simulink model "newattempt01"  (R2020a)
settings: Solver=FixedStepAuto  StartTime=0.0  StopTime=0.02  FixedStep=0.00001  RelTol=1e-3
model workspace (MAT data in the model file):
  K_Spring = 3
  R = 7
  V = 350
  V_T = Simulink.Parameter
  V_T.Value = 350
  V_T.DataType = 'auto'
  V_T.Dimensions = [1 1]
libraries: nesl_utility x27, fl_lib x21, sdl_lib x1
settings Model: OrderedModelArguments=off  Creator=insat  LastModifiedBy=insat

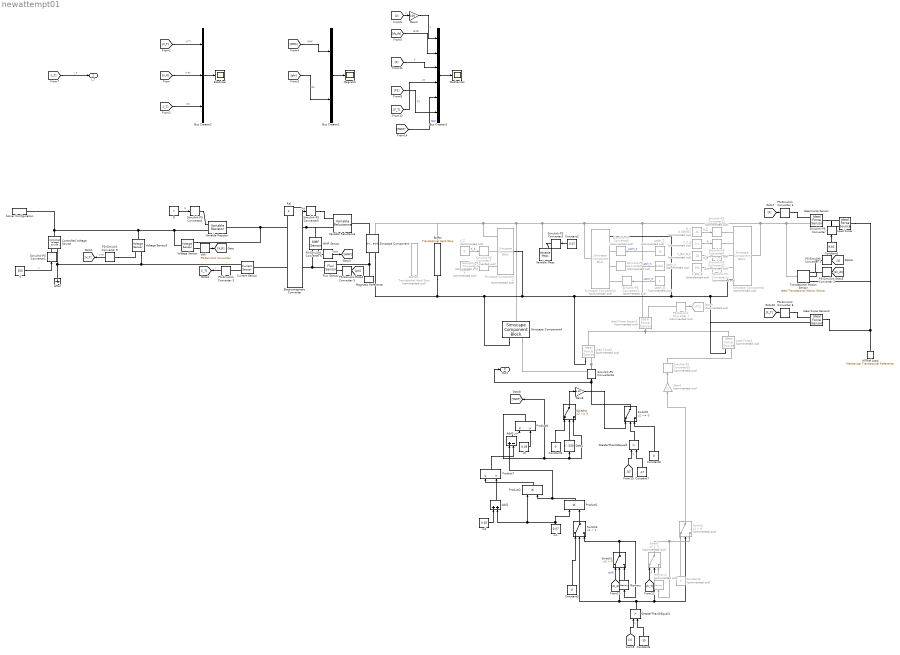
== system newattempt01 ==
  Add1 : Sum
  Add2 : Sum  Inputs=+-
  Buffer : fl_lib/Mechanical/Translational Elements/Translational Hard Stop  upper_bnd=20 mm  lower_bnd=-.9 mm  stiff_up=100 N/mm  stiff_low=100 N/mm  D_up=100 s*N/mm  D_low=100 s*N/mm  model=simscape.enum.hardstop.fullundamped  transition=1 mm  v_specify=off  v_priority=None  v=0 m/s  v_nominal_specify=off  v_nominal_unit=m/s  v_nominal_value=1  f_specify=off  f_priority=None  f=0 N  f_nominal_specify=off  f_nominal_unit=N  f_nominal_value=1  x_specify=off  x_priority=High  x=0 m  x_nominal_specify=off  x_nominal_unit=m  x_nominal_value=1
  Buffer1 : fl_lib/Mechanical/Translational Elements/Translational Hard Stop  Commented=on  upper_bnd=20 mm  lower_bnd=-.9 mm  stiff_up=10000 N/mm  stiff_low=10000 N/mm  D_up=0.7 s*N/mm  D_low=0.7 s*N/mm  model=simscape.enum.hardstop.fullundamped  transition=1 mm  v_specify=off  v_priority=None  v=0 m/s  v_nominal_specify=off  v_nominal_unit=m/s  v_nominal_value=1  f_specify=off  f_priority=None  f=0 N  f_nominal_specify=off  f_nominal_unit=N  f_nominal_value=1  x_specify=off  x_priority=High  x=0 m  x_nominal_specify=off  x_nominal_unit=m  x_nominal_value=1
  Bus Creator1 : BusCreator  Inputs=2
  Bus Creator2 : BusCreator  Inputs=3
  Bus Creator3 : BusCreator  Inputs=6
  Constant1 : Constant  Value=9.81
  Constant2 : Constant  Value=0.07
  Constant3 : Constant  Commented=on  Value=0
  Constant4 : Constant  Value=-15
  Constant5 : Constant  Value=0
  Constant6 : Constant  Value=0
  Constant7 : Constant  Value=-17
  Constant8 : Constant  Value=0
  Controlled Voltage Source : fl_lib/Electrical/Electrical Sources/Controlled Voltage Source
  Current Sensor : fl_lib/Electrical/Electrical Sensors/Current Sensor
  D_V : Constant  Commented=on  Value=0.000001
  Delay : Delay  DelayLength=250  InitialCondition=0  UseCircularBuffer=on
  ERef : fl_lib/Electrical/Electrical Elements/Electrical Reference
  Electrical : Scope
  Electromagnetic Converter : fl_lib/Magnetic/Magnetic Elements/Electromagnetic Converter  Nw=1000  i_specify=off  i_priority=None  i=0 A  i_nominal_specify=off  i_nominal_unit=A  i_nominal_value=1  v_specify=off  v_priority=None  v=0 V  v_nominal_specify=off  v_nominal_unit=V  v_nominal_value=1  mmf_specify=off  mmf_priority=None  mmf=0 A  mmf_nominal_specify=off  mmf_nominal_unit=A  mmf_nominal_value=1  phi_specify=off  phi_priority=High  phi=0 Wb  phi_nominal_specify=off  phi_nominal_unit=Wb  phi_nominal_value=1
      settings: SourceProductBaseCode=SS  InternalSimscapePortConfiguration="{\"Bottom\":[],\"Left\":[{\"id\":\"p\",\"label\":\"+\",\"type\":\"foundation.electrical.electrical\"},{\"id\":\"n\",\"label\":\"-\",\"type\":\"foundation.electrical.electrical\"}],\"Right\":[{\"id\":\"N\",\"label\":\"N\",\"type\":\"foundation.magnetic.magnetic\"},{\"id\":\"S\",\"label\":\"S\",\"type\":\"foundation.magnetic.magnetic\"}],\"Top\":[]}"
  F_BW_B : Constant  Commented=on  Value=250
  F_C_B : Constant  Commented=on  Value=0.1
  Flux Sensor : fl_lib/Magnetic/Magnetic Sensors/Flux Sensor
      settings: SourceProductBaseCode=SS  InternalSimscapePortConfiguration="{\"Bottom\":[],\"Left\":[{\"id\":\"N\",\"label\":\"N\",\"type\":\"foundation.magnetic.magnetic\"}],\"Right\":[{\"id\":\"PHI\",\"label\":\"\",\"type\":\"output\"},{\"id\":\"S\",\"label\":\"S\",\"type\":\"foundation.magnetic.magnetic\"}],\"Top\":[]}"
  Gain2 : Gain  Gain=100
  Gain3 : Gain  Gain=-0.05
  Gain4 : Gain  Commented=on  Gain=-1
  Goto9 : Goto  Commented=on  GotoTag=F2
  GreaterThanOrEqual1 : RelationalOperator  Operator=>  OutDataTypeStr=boolean  ZeroCross=off  RndMeth=Simplest
  GreaterThanOrEqual2 : RelationalOperator  Operator=>  OutDataTypeStr=boolean  ZeroCross=off  RndMeth=Simplest
  Ideal Force Sensor : fl_lib/Mechanical/Mechanical Sensors/Ideal Force Sensor
  Ideal Force Sensor1 : fl_lib/Mechanical/Mechanical Sensors/Ideal Force Sensor  Commented=on
  Ideal Force Sensor2 : fl_lib/Mechanical/Mechanical Sensors/Ideal Force Sensor
  K : Constant  Commented=on  Value=3
  K_Z : Constant  Commented=on  Value=0
  Latch_D : Constant  Commented=on
  Latch_K : Constant  Commented=on  Value=0.0001
  Latch_Z : Constant  Commented=on  Value=15
  Load Force : fl_lib/Mechanical/Mechanical Sources/Ideal Force Source
  Load Force1 : fl_lib/Mechanical/Mechanical Sources/Ideal Force Source  Commented=on
  Load Force2 : fl_lib/Mechanical/Mechanical Sources/Ideal Force Source  Commented=on
  MMF Sensor : fl_lib/Magnetic/Magnetic Sensors/MMF Sensor
      settings: SourceProductBaseCode=SS  InternalSimscapePortConfiguration="{\"Bottom\":[],\"Left\":[{\"id\":\"N\",\"label\":\"N\",\"type\":\"foundation.magnetic.magnetic\"}],\"Right\":[{\"id\":\"MMF\",\"label\":\"\",\"type\":\"output\"},{\"id\":\"S\",\"label\":\"S\",\"type\":\"foundation.magnetic.magnetic\"}],\"Top\":[]}"
  MTRef Load : fl_lib/Mechanical/Translational Elements/Mechanical Translational Reference
  Magnetic : Scope
  Magnetic Reference : fl_lib/Magnetic/Magnetic Elements/Magnetic Reference
      settings: SourceProductBaseCode=SS  InternalSimscapePortConfiguration="{\"Bottom\":[],\"Left\":[{\"id\":\"M\",\"label\":\"\",\"type\":\"foundation.magnetic.magnetic\"}],\"Right\":[],\"Top\":[]}"
  Mechanical : Scope
  Memory : Memory
  Memory1 : Memory  Commented=on
  PS-Simulink Converter 1 : nesl_utility/PS-Simulink Converter  PhysicalDomain=network_engine_domain  SubClassName=ps_output  LeftPortType=input  RightPortType=output  PseudoPeriodic=off  Frequencies=[]  Unit=mm  AffineConversion=off
  PS-Simulink Converter 2 : nesl_utility/PS-Simulink Converter  PhysicalDomain=network_engine_domain  SubClassName=ps_output  LeftPortType=input  RightPortType=output  PseudoPeriodic=off  Frequencies=[]  Unit=mm/s  AffineConversion=off
  PS-Simulink Converter 3 : nesl_utility/PS-Simulink Converter  PhysicalDomain=network_engine_domain  SubClassName=ps_output  LeftPortType=input  RightPortType=output  PseudoPeriodic=off  Frequencies=[]  Unit=A  AffineConversion=off
  PS-Simulink Converter 4 : nesl_utility/PS-Simulink Converter  PhysicalDomain=network_engine_domain  SubClassName=ps_output  LeftPortType=input  RightPortType=output  PseudoPeriodic=off  Frequencies=[]  Unit=N  AffineConversion=off
  PS-Simulink Converter 5 : nesl_utility/PS-Simulink Converter  PhysicalDomain=network_engine_domain  SubClassName=ps_output  LeftPortType=input  RightPortType=output  PseudoPeriodic=off  Frequencies=[]  Unit=Wb  AffineConversion=off
  PS-Simulink Converter 6 : nesl_utility/PS-Simulink Converter  PhysicalDomain=network_engine_domain  SubClassName=ps_output  LeftPortType=input  RightPortType=output  PseudoPeriodic=off  Frequencies=[]  Unit=A  AffineConversion=off
  PS-Simulink Converter 7 : nesl_utility/PS-Simulink Converter  Commented=on  PhysicalDomain=network_engine_domain  SubClassName=ps_output  LeftPortType=input  RightPortType=output  PseudoPeriodic=off  Frequencies=[]  Unit=N  AffineConversion=off
  PS-Simulink Converter 8 : nesl_utility/PS-Simulink Converter  PhysicalDomain=network_engine_domain  SubClassName=ps_output  LeftPortType=input  RightPortType=output  PseudoPeriodic=off  Frequencies=[]  Unit=N  AffineConversion=off
  PS-Simulink Converter 9 : nesl_utility/PS-Simulink Converter  PhysicalDomain=network_engine_domain  SubClassName=ps_output  LeftPortType=input  RightPortType=output  PseudoPeriodic=off  Frequencies=[]  Unit=V  AffineConversion=off
  Product1 : Product  Inputs=**
  Product2 : Product  Inputs=**
  Product7 : Product  Inputs=*/
  Product8 : Product  Inputs=*/
  R : Constant  Value=7
  Rel : Constant
  Simscape Component : SimscapeComponentBlock  SourceFile=reluctance_force_actuator_modified  ComponentPath=reluctance_force_actuator_modified  ComponentVariants="[\"reluctance_force_actuator_modified\"]"  ComponentVariantNames="[\"reluctance_force_actuator_modified\"]"  ClassName=reluctance_force_actuator_modified  SchemaVersion=1  x0=30 mm  xbffr=1 mm  CSA=1.7671 cm^2  mur=1  K_contact=500 N/mm  D_contact=0.2 s*N/mm  mmf_specify=off  mmf_priority=None  mmf=0 A  mmf_nominal_specify=off  mmf_nominal_unit=A  mmf_nominal_value=1  phi_specify=off  phi_priority=None  phi=0 Wb  phi_nominal_specify=off  phi_nominal_unit=Wb  phi_nominal_value=1  f_specify=off  f_priority=None  f=0 N  f_nominal_specify=off  f_nominal_unit=N  f_nominal_value=1  u_specify=off  u_priority=None  u=0 m/s  u_nominal_specify=off  u_nominal_unit=m/s  u_nominal_value=1
      settings: CopyFcn=simscape.engine.sli.internal.componentblockcallback(gcbh,'COPY')  PreCopyFcn=simscape.engine.sli.internal.componentblockcallback(gcbh,'PRECOPY')  PreDeleteFcn=simscape.engine.sli.internal.componentblockcallback(gcbh,'PREDELETE')  InternalSimscapePortConfiguration="{\"Bottom\":[],\"Left\":[{\"id\":\"N\",\"label\":\"N\",\"type\":\"foundation.magnetic.magnetic\"},{\"id\":\"R\",\"label\":\"R\",\"type\":\"foundation.mechanical.translational.translational\"}],\"Right\":[{\"id\":\"S\",\"label\":\"S\",\"type\":\"foundation.magnetic.magnetic\"},{\"id\":\"C\",\"label\":\"C\",\"type\":\"foundation.mechanical.translational.translational\"}],\"Top\":[]}"
      mask Type: Reluctance Force Actuator
  Simscape Component1 : SimscapeComponentBlock  Commented=on  SourceFile=mechanical_forces_from_reluctance_force_actuator  ComponentPath=mechanical_forces_from_reluctance_force_actuator  ComponentVariants="[\"mechanical_forces_from_reluctance_force_actuator\"]"  ComponentVariantNames="[\"mechanical_forces_from_reluctance_force_actuator\"]"  ClassName=mechanical_forces_from_reluctance_force_actuator  SchemaVersion=1  latch_dur=1 mm  transition=0.1 mm  v_specify=off  v_priority=None  v=0 m/s  v_nominal_specify=off  v_nominal_unit=m/s  v_nominal_value=1  f_specify=off  f_priority=None  f=0 N  f_nominal_specify=off  f_nominal_unit=N  f_nominal_value=1  x_specify=off  x_priority=High  x=0 m  x_nominal_specify=off  x_nominal_unit=m  x_nominal_value=1
      settings: CopyFcn=simscape.engine.sli.internal.componentblockcallback(gcbh,'COPY')  PreCopyFcn=simscape.engine.sli.internal.componentblockcallback(gcbh,'PRECOPY')  PreDeleteFcn=simscape.engine.sli.internal.componentblockcallback(gcbh,'PREDELETE')  InternalSimscapePortConfiguration="{\"Bottom\":[],\"Left\":[{\"id\":\"R\",\"label\":\"R\",\"type\":\"foundation.mechanical.translational.translational\"},{\"id\":\"latch_loc\",\"label\":\"Z\",\"type\":\"input\"},{\"id\":\"K_latch\",\"label\":\"K\",\"type\":\"input\"},{\"id\":\"D_latch\",\"label\":\"D\",\"type\":\"input\"}],\"Right\":[{\"id\":\"C\",\"label\":\"C\",\"type\":\"foundation.mechanical.translational.translational\"}],\"Top\":[]}"
      mask Type: Mechanical Forces from Reluctance Force Actuator
  Simscape Component2 : SimscapeComponentBlock  Commented=on  SourceFile=var_trans_spring_mod  ComponentPath=var_trans_spring_mod  ComponentVariants="[\"var_trans_spring_mod\"]"  ComponentVariantNames="[\"var_trans_spring_mod\"]"  ClassName=var_trans_spring_mod  SchemaVersion=1  Kmin=1 N/m
      settings: CopyFcn=simscape.engine.sli.internal.componentblockcallback(gcbh,'COPY')  PreCopyFcn=simscape.engine.sli.internal.componentblockcallback(gcbh,'PRECOPY')  PreDeleteFcn=simscape.engine.sli.internal.componentblockcallback(gcbh,'PREDELETE')  InternalSimscapePortConfiguration="{\"Bottom\":[],\"Left\":[{\"id\":\"R\",\"label\":\"R\",\"type\":\"foundation.mechanical.translational.translational\"}],\"Right\":[{\"id\":\"K\",\"label\":\"K\",\"type\":\"input\"},{\"id\":\"Z\",\"label\":\"Z\",\"type\":\"input\"},{\"id\":\"C\",\"label\":\"C\",\"type\":\"foundation.mechanical.translational.translational\"}],\"Top\":[]}"
      mask Type: Variable Translational Spring
  Simscape Component3 : SimscapeComponentBlock  Commented=on  SourceFile=friction_var  ComponentPath=friction_var  ComponentVariants="[\"friction_var\"]"  ComponentVariantNames="[\"friction_var\"]"  ClassName=friction_var  SchemaVersion=1  v_specify=off  v_priority=None  v=0 m/s  v_nominal_specify=off  v_nominal_unit=m/s  v_nominal_value=1  f_specify=off  f_priority=None  f=0 N  f_nominal_specify=off  f_nominal_unit=N  f_nominal_value=1
      settings: CopyFcn=simscape.engine.sli.internal.componentblockcallback(gcbh,'COPY')  PreCopyFcn=simscape.engine.sli.internal.componentblockcallback(gcbh,'PRECOPY')  PreDeleteFcn=simscape.engine.sli.internal.componentblockcallback(gcbh,'PREDELETE')  InternalSimscapePortConfiguration="{\"Bottom\":[],\"Left\":[{\"id\":\"R\",\"label\":\"R\",\"type\":\"foundation.mechanical.translational.translational\"},{\"id\":\"brkwy_frc\",\"label\":\"F_BW_B\",\"type\":\"input\"},{\"id\":\"brkwy_vel\",\"label\":\"V_BW_B\",\"type\":\"input\"},{\"id\":\"Col_frc\",\"label\":\"F_C_B\",\"type\":\"input\"},{\"id\":\"visc_coef\",\"label\":\"D_V\",\"type\":\"input\"}],\"Right\":[{\"id\":\"C\",\"label\":\"C\",\"type\":\"foundation.mechanical.translational.translational\"}],\"Top\":[]}"
      mask Type: Translational Friction Controllable
  Simscape Component4 : SimscapeComponentBlock  SourceFile=damper_mod  ComponentPath=damper_mod  ComponentVariants="[\"damper_mod\"]"  ComponentVariantNames="[\"damper_mod\"]"  ClassName=damper_mod  SchemaVersion=1  v_specify=off  v_priority=None  v=0 m/s  v_nominal_specify=off  v_nominal_unit=m/s  v_nominal_value=1  f_specify=off  f_priority=None  f=0 N  f_nominal_specify=off  f_nominal_unit=N  f_nominal_value=1
      settings: CopyFcn=simscape.engine.sli.internal.componentblockcallback(gcbh,'COPY')  PreCopyFcn=simscape.engine.sli.internal.componentblockcallback(gcbh,'PRECOPY')  PreDeleteFcn=simscape.engine.sli.internal.componentblockcallback(gcbh,'PREDELETE')  InternalSimscapePortConfiguration="{\"Bottom\":[],\"Left\":[{\"id\":\"R\",\"label\":\"R\",\"type\":\"foundation.mechanical.translational.translational\"},{\"id\":\"D\",\"label\":\"Damping coefficient\",\"type\":\"input\"}],\"Right\":[{\"id\":\"C\",\"label\":\"C\",\"type\":\"foundation.mechanical.translational.translational\"}],\"Top\":[]}"
      mask Type: Translational Damper
  Simulink-PS Converter{,1,3..5,16} (6 alike) : nesl_utility/Simulink-PS Converter  PhysicalDomain=network_engine_domain  SubClassName=ps_input  LeftPortType=input  RightPortType=output  PseudoPeriodic=off  Frequencies=[]  NoiseDistribution=none  NoiseParameters=[]  Unit=1  AffineConversion=off  FilteringAndDerivatives=zero  SimscapeFilterOrder=1  InputFilterTimeConstant=.001  UdotUserProvided=0
  Simulink-PS Converter{2,6..13,15} (10 alike) : nesl_utility/Simulink-PS Converter  Commented=on  PhysicalDomain=network_engine_domain  SubClassName=ps_input  LeftPortType=input  RightPortType=output  PseudoPeriodic=off  Frequencies=[]  NoiseDistribution=none  NoiseParameters=[]  Unit=1  AffineConversion=off  FilteringAndDerivatives=zero  SimscapeFilterOrder=1  InputFilterTimeConstant=.001  UdotUserProvided=0
  Solver Configuration : nesl_utility/Solver Configuration  PhysicalDomain=network_engine_domain  SubClassName=solver  LeftPortType=input  RightPortType=generic  Tones=[]  Harmonics=[]  SimulateNoise=off  Profile=off  UseLocalSampling=off  EnableSwitchedLinearOptims=on  FrequencyDomain=off  UseCCode=off  RelTol=0.001  AbsTol=1e-06  MinStep=1e-09  ToWorkspace=off  RevertToSquareIcSolve=off  NumHomotopyIterations=100  PhasorMode=off  PhasorModeNumHarmonics=1  DoDC=off  ResidualTolerance=1e-9  UseLocalSolver=off  LocalSolverChoice=NE_BACKWARD_EULER_ADVANCER  LocalSolverSampleTime=.001  DoFixedCost=off  MaxNonlinIter=3  MaxModeIter=2  LinearAlgebra=auto  EquationFormulation=NE_TIME_EF  DelaysMemoryBudget=1024  AutomaticFiltering=on  FilteringTimeConstant=0.0001  PartitionStorageMethod=AS_NEEDED  PartitionMemoryBudget=1024  PartitionMethod=FAST
  Switch : Switch  Commented=on  Criteria=u2 > Threshold
  Switch1 : Switch  Criteria=u2 > Threshold
  Switch2 : Switch  Commented=on  Criteria=u2 > Threshold
  Switch3 : Switch  Criteria=u2 > Threshold
  Switch4 : Switch  Criteria=u2 ~= 0  ZeroCross=off
  Switch5 : Switch  Criteria=u2 ~= 0  ZeroCross=off
  Translational Motion Sensor : fl_lib/Mechanical/Mechanical Sensors/Ideal Translational Motion Sensor  offset=0 mm
  V : Constant  Value=350
  V(R) : nesl_utility/PS-Simulink Converter  PhysicalDomain=network_engine_domain  SubClassName=ps_output  LeftPortType=input  RightPortType=output  PseudoPeriodic=off  Frequencies=[]  Unit=V  AffineConversion=off
  V_BW_B_C : Constant  Commented=on  Value=10
  Variable Mass : sdl_lib/Inertias & Loads/Variable Mass  minimum_mass=0.0001 kg  p_specify=off  p_priority=High  p=0 m*kg/s  p_nominal_specify=off  p_nominal_unit=m*kg/s  p_nominal_value=1
      settings: SourceProductBaseCode=LD  InternalSimscapePortConfiguration="{\"Bottom\":[],\"Left\":[{\"id\":\"M\",\"label\":\"\",\"type\":\"input\"},{\"id\":\"A\",\"label\":\"\",\"type\":\"foundation.mechanical.translational.translational\"}],\"Right\":[],\"Top\":[]}"
  Variable Reluctance : fl_lib/Magnetic/Magnetic Elements/Variable Reluctance  Xmin=1 m  CSA=1 m^2  mur=1  phi_specify=off  phi_priority=None  phi=0 Wb  phi_nominal_specify=off  phi_nominal_unit=Wb  phi_nominal_value=1  mmf_specify=off  mmf_priority=None  mmf=0 A  mmf_nominal_specify=off  mmf_nominal_unit=A  mmf_nominal_value=1
      settings: SourceProductBaseCode=SS  InternalSimscapePortConfiguration="{\"Bottom\":[],\"Left\":[{\"id\":\"N\",\"label\":\"N\",\"type\":\"foundation.magnetic.magnetic\"},{\"id\":\"X\",\"label\":\"\",\"type\":\"input\"}],\"Right\":[{\"id\":\"S\",\"label\":\"S\",\"type\":\"foundation.magnetic.magnetic\"}],\"Top\":[]}"
  Variable Resistor : fl_lib/Electrical/Electrical Elements/Variable Resistor  Rmin=0 Ohm  i_specify=off  i_priority=None  i=0 A  i_nominal_specify=off  i_nominal_unit=A  i_nominal_value=1  v_specify=off  v_priority=None  v=0 V  v_nominal_specify=off  v_nominal_unit=V  v_nominal_value=1
  Voltage Sensor : fl_lib/Electrical/Electrical Sensors/Voltage Sensor
  Voltage Sensor3 : fl_lib/Electrical/Electrical Sensors/Voltage Sensor
  dt : Constant  Value=0.05
  m1 : Constant  Value=0.07
  m2 : Constant  Value=0.35
  i_T : Outport  SignalName=i_T
  Out1 : Outport  Port=2
  wires:
  PS-Simulink Converter 5/1 -> [phi]
  PS-Simulink Converter 6/1 -> [MMF]  "MMF"
  PS-Simulink Converter 9/1 -> [V_T]  "V(T)"
  PS-Simulink Converter 3/1 -> [i_T]  "i"
  PS-Simulink Converter 1/1 -> [z]
  V(R)/1 -> [V_R]
  PS-Simulink Converter 2/1 -> [dz_dt]
  [V_R] -> Bus Creator2/2  "V(R)"
  [V_T] -> Bus Creator2/1  "V(T)"
  Bus Creator2/1 -> Electrical/1
  [i_T] -> Bus Creator2/3  "i(T)"
  Bus Creator1/1 -> Magnetic/1
  [MMF] -> Bus Creator1/1  "MMF"
  [phi] -> Bus Creator1/2  "phi"
  Bus Creator3/1 -> Mechanical/1
  [z] -> Gain2/1  "z"
  [dz_dt] -> Bus Creator3/2  "dz/dt"
  Constant1/1 -> Simulink-PS Converter/1
  [F] -> Bus Creator3/3  "F"
  Constant2/1 -> Simulink-PS Converter3/1
  K/1 -> Simulink-PS Converter2/1  "K"
  R/1 -> Simulink-PS Converter4/1  "R"
  Rel/1 -> Simulink-PS Converter5/1  "Rel"
  K_Z/1 -> Simulink-PS Converter7/1  "K_Z"
  Latch_Z/1 -> Simulink-PS Converter8/1  "Latch_Z"
  Latch_K/1 -> Simulink-PS Converter9/1  "Latch_K"
  Latch_D/1 -> Simulink-PS Converter10/1  "Latch_D"
  F_C_B/1 -> Simulink-PS Converter6/1  "K"
  D_V/1 -> Simulink-PS Converter11/1  "K_Z"
  F_BW_B/1 -> Simulink-PS Converter13/1  "K"
  V_BW_B_C/1 -> Simulink-PS Converter12/1  "K_Z"
  V/1 -> Simulink-PS Converter1/1  "V"
  [i_T] -> i_T/1  "i_T"
  [F2] -> Bus Creator3/6  "F2"
  Memory/1 -> Switch1/3
  Constant3/1 -> Switch2/1
  Constant4/1 -> GreaterThanOrEqual1/2
  [z] -> GreaterThanOrEqual1/1  "z"
  GreaterThanOrEqual1/1 -> Switch2/2, Switch/2, Switch3/2, Switch1/2
  [F_T] -> Switch/1  "F"
  Constant5/1 -> Switch3/1
  [dz_dt] -> Switch1/1  "dz/dt"
  Memory1/1 -> Switch/3
  Switch1/1 -> Switch3/3, Memory/1
  PS-Simulink Converter 4/1 -> [F]
  Switch/1 -> Memory1/1, Switch2/3
  Switch2/1 -> Gain4/1
  PS-Simulink Converter 7/1 -> Goto9/1
  PS-Simulink Converter 8/1 -> [F_T]
  [F_T] -> Bus Creator3/4  "FT"
  Delay/1 -> Switch4/2
  Constant6/1 -> Switch4/1
  Gain2/1 -> Bus Creator3/1  "z"
  Gain4/1 -> Simulink-PS Converter15/1
  [TEST] -> Bus Creator3/5  "TEST"
  Gain3/1 -> Switch5/1
  Switch4/1 -> Gain3/1
  m1/1 -> Add1/2, Product2/1, Product1/1
  Switch3/1 -> Product1/2
  Product1/1 -> Product2/2, Add2/1
  Product2/1 -> Product7/1
  m2/1 -> Add1/1
  Add1/1 -> Product7/2
  dt/1 -> Product8/2
  Product7/1 -> Add2/2
  Product8/1 -> [TEST], Switch4/3, Delay/1
  Add2/1 -> Product8/1
  Constant7/1 -> GreaterThanOrEqual2/2
  [z] -> GreaterThanOrEqual2/1  "z"
  GreaterThanOrEqual2/1 -> Switch5/2
  Constant8/1 -> Switch5/3
  Switch5/1 -> Out1/1, Simulink-PS Converter16/1
  connections:
  Voltage Sensor/RConn2 -- Variable Resistor/RConn1 -- Electromagnetic Converter/LConn1
  Flux Sensor/RConn2 -- Simscape Component/RConn1 -- Magnetic Reference/LConn1
  Electromagnetic Converter/RConn1 -- Variable Reluctance/LConn1 -- MMF Sensor/LConn1
  Simulink-PS Converter1/RConn1 -- Controlled Voltage Source/RConn1
  Current Sensor/RConn2 -- Voltage Sensor3/RConn2 -- Controlled Voltage Source/RConn2 -- ERef/LConn1
  Electromagnetic Converter/LConn2 -- Current Sensor/LConn1
  Flux Sensor/LConn1 -- MMF Sensor/RConn2 -- Electromagnetic Converter/RConn2
  Translational Motion Sensor/RConn3 -- PS-Simulink Converter 1/LConn1
  PS-Simulink Converter 9/LConn1 -- Voltage Sensor3/RConn1
  Voltage Sensor/RConn1 -- V(R)/LConn1
  PS-Simulink Converter 6/LConn1 -- MMF Sensor/RConn1
  PS-Simulink Converter 2/LConn1 -- Translational Motion Sensor/RConn2
  Current Sensor/RConn1 -- PS-Simulink Converter 3/LConn1
  Simscape Component/LConn1 -- Variable Reluctance/RConn1
  Flux Sensor/RConn1 -- PS-Simulink Converter 5/LConn1
  Simulink-PS Converter/RConn1 -- Load Force/RConn1
  Voltage Sensor/LConn1 -- Controlled Voltage Source/LConn1 -- Solver Configuration/RConn1 -- Voltage Sensor3/LConn1 -- Variable Resistor/LConn2
  Simulink-PS Converter3/RConn1 -- Variable Mass/LConn1
  Simulink-PS Converter4/RConn1 -- Variable Resistor/LConn1
  Simulink-PS Converter5/RConn1 -- Variable Reluctance/LConn2
  Simscape Component2/RConn1 -- Simulink-PS Converter2/RConn1
  Simscape Component2/RConn2 -- Simulink-PS Converter7/RConn1
  Simulink-PS Converter8/RConn1 -- Simscape Component1/LConn2
  Simulink-PS Converter9/RConn1 -- Simscape Component1/LConn3
  Simscape Component1/LConn4 -- Simulink-PS Converter10/RConn1
  Simulink-PS Converter6/RConn1 -- Simscape Component3/LConn4
  Simulink-PS Converter11/RConn1 -- Simscape Component3/LConn5
  Simulink-PS Converter13/RConn1 -- Simscape Component3/LConn2
  Simscape Component3/LConn3 -- Simulink-PS Converter12/RConn1
  Load Force2/RConn1 -- Simscape Component4/LConn2 -- Simulink-PS Converter16/RConn1
  Load Force1/RConn1 -- Simulink-PS Converter15/RConn1
  PS-Simulink Converter 4/LConn1 -- Ideal Force Sensor/RConn2
  Simscape Component1/RConn1 -- Simscape Component4/RConn1 -- Simscape Component/LConn2 -- Buffer/RConn1 -- Simscape Component2/RConn3 -- Variable Mass/LConn2 -- Translational Motion Sensor/LConn1 -- Ideal Force Sensor/RConn1 -- Simscape Component3/RConn1 -- Ideal Force Sensor1/RConn1
  Ideal Force Sensor/LConn1 -- Load Force/RConn2
  PS-Simulink Converter 7/LConn1 -- Ideal Force Sensor1/RConn2
  Ideal Force Sensor1/LConn1 -- Load Force1/LConn1 -- Load Force2/LConn1
  PS-Simulink Converter 8/LConn1 -- Ideal Force Sensor2/RConn2
  Buffer/LConn1 -- Simscape Component/RConn2 -- Simscape Component4/LConn1 -- Simscape Component2/LConn1 -- Load Force2/RConn2 -- Ideal Force Sensor2/RConn1 -- Load Force1/RConn2 -- Simscape Component3/LConn1 -- Simscape Component1/LConn1
  Ideal Force Sensor2/LConn1 -- MTRef Load/LConn1 -- Load Force/LConn1 -- Translational Motion Sensor/RConn1
